simulink model "servo_sim"  (Simulink 7.1)
settings: Solver=FixedStepDiscrete  StartTime=0.0  StopTime=60  RelTol=1e-3
libraries: arduino_io_lib x4, simulink x1
settings Model: Creator=gcampa  LastModifiedBy=gcampa
settings OptimizationCC: InitFltsAndDblsToZero=off
settings DebuggingCC: StrictBusMsg=ErrorLevel1
settings GRTTargetCC: CPPClassGenCompliant=off

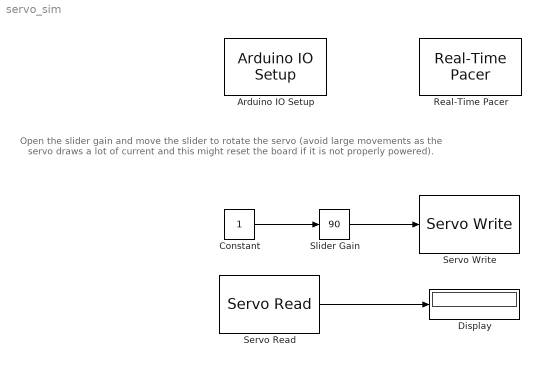
== system servo_sim ==
  note: Open the slider gain and move the slider to rotate the servo
      | (avoid large movements as the servo draws a lot of current
      | and this might reset the board if it is not properly powered).
  Arduino IO Setup : arduino_io_lib/Arduino IO Setup  Priority=3  arduinoVar=Arduino1  comPort=COM9
  Constant : Constant
  Display : Display
  Real-Time Pacer : arduino_io_lib/Real-Time Pacer  simTimePerRealTime=1
  Servo Read : arduino_io_lib/Servo Read  arduinoVar=Arduino1  servoNum=1  T=0.2
  Servo Write : arduino_io_lib/Servo Write  arduinoVar=Arduino1  servoNum=1  T=0.2
  Slider Gain : simulink/Math Operations/Slider Gain  SystemSampleTime=-1  low=10  gain=90  high=170
  wires:
  Constant/1 -> Slider Gain/1
  Servo Read/1 -> Display/1
  Slider Gain/1 -> Servo Write/1
